simulink model "Microinverter_Paper_Model_MK_2018a"  (R2018a)
settings: Solver=FixedStepDiscrete  StartTime=0.0  StopTime=0.3  RelTol=1e-3
undefined symbols (not defined in the file): sigbuilder_block
libraries: powerlib x53, simulink x5, powerlib_meascontrol x4, re_lib x1
settings Model: Creator=jasil  LastModifiedBy=mwkane
settings SFSimCC: SimUseLocalCustomCode=on
settings RTWCC: RTWUseLocalCustomCode=on
settings CodeAppCC: StateflowObjectComments=on

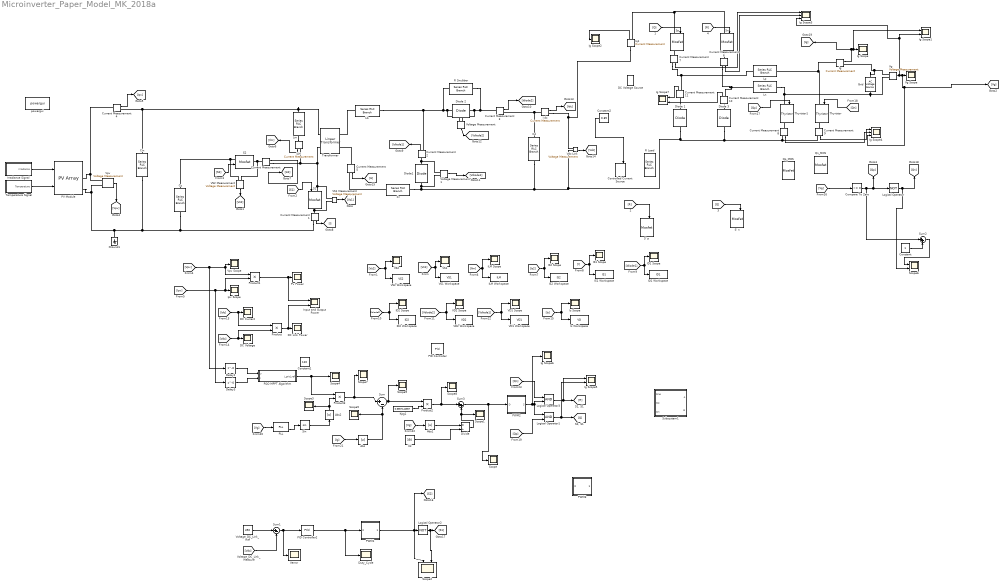
== system Microinverter_Paper_Model_MK_2018a ==
  Abs : Abs
  Abs1 : Abs
  Abs2 : Abs
  Cc : powerlib/Elements/Series RLC Branch  LConnTagsString=__new0  RConnTagsString=__new0  BranchType=RC  Resistance=0.000001  Inductance=1e-3  SetiL0=off  InitialCurrent=0  Capacitance=2.2e-6  Setx0=off  InitialVoltage=0  Measurements=None
      settings: SourceProductName=Simscape Electrical
  Cd : powerlib/Elements/Series RLC Branch  LConnTagsString=__new0  RConnTagsString=__new0  BranchType=RC  Resistance=0.000001  Inductance=1e-3  SetiL0=off  InitialCurrent=0  Capacitance=1  Setx0=off  InitialVoltage=0  Measurements=None
      settings: SourceProductName=Simscape Electrical
  Cin : powerlib/Elements/Series RLC Branch  LConnTagsString=__new0  RConnTagsString=__new0  BranchType=RC  Resistance=0.000001  Inductance=1e-3  SetiL0=off  InitialCurrent=0  Capacitance=1e-3  Setx0=off  InitialVoltage=0  Measurements=Branch voltage
      settings: SourceProductName=Simscape Electrical
  Compare To Zero : simulink/Logic and Bit Operations/Compare To Zero  relop=>=  OutDataTypeStr=boolean
  Constant : Constant
  Constant1 : Constant  Value=120
  Constant2 : Constant  Value=0.85
  Controlled Current Source : powerlib/Electrical Sources/Controlled Current Source  Initialize=on  Source_Type=AC  Amplitude=0  Phase=0  Frequency=0  Measurements=None
      settings: SourceProductName=Simscape Electrical
  Cr : powerlib/Elements/Series RLC Branch  LConnTagsString=__new0  RConnTagsString=__new0  BranchType=RC  Resistance=0.000001  Inductance=1e-3  SetiL0=off  InitialCurrent=0  Capacitance=2.4e-6  Setx0=off  InitialVoltage=0  Measurements=None
      settings: SourceProductName=Simscape Electrical
  Current Measurement{,1..11} (12 alike) : powerlib/Measurements/Current Measurement  PhasorSimulation=off  OutputType=Complex  PSBequivalent=0
      settings: SourceProductName=Simscape Electrical
  DC Current : Scope
  DC Link Power : Scope
  DC Voltage : Scope
  DC Voltage Source : powerlib/Electrical Sources/DC Voltage Source  Amplitude=350  Measurements=None
      settings: SourceProductName=Simscape Electrical
  Delay2 : Delay  DelayLength=0  SampleTime=0.0001
  Delay3 : Delay  DelayLength=0  SampleTime=0.0001
  Diode 1 : powerlib/Power Electronics/Diode  Ron=1  Lon=0  Vf=0.8  IC=0  UseSnubber=0  Rs=1e5  Cs=inf  Measurements=off
      settings: SourceProductName=Simscape Electrical
  Diode 2 : powerlib/Power Electronics/Diode  Ron=1  Lon=0  Vf=0.8  IC=0  UseSnubber=0  Rs=inf  Cs=0  Measurements=off
      settings: SourceProductName=Simscape Electrical
  Diode 3 : powerlib/Power Electronics/Diode  Ron=1  Lon=0  Vf=0.8  IC=0  UseSnubber=0  Rs=1e5  Cs=inf  Measurements=off
      settings: SourceProductName=Simscape Electrical
  Diode1 : powerlib/Power Electronics/Diode  Ron=0.01  Lon=0  Vf=0.8  IC=0  UseSnubber=0  Rs=inf  Cs=0  Measurements=off
      settings: SourceProductName=Simscape Electrical
  Divide : Product  Inputs=*/
  Duty_Cycle : Scope
  Grid : powerlib/Electrical Sources/AC Voltage Source  Amplitude=311.126  Phase=0  Frequency=60  SampleTime=0  Measurements=None  BusType=swing  Pref=0  Qref=0  Qmin=-inf  Qmax=+inf
      settings: SourceProductName=Simscape Electrical
  Ground1 : powerlib/Elements/Ground  LConnTagsString=a
      settings: SourceProductName=Simscape Electrical
  I dc : powerlib/Measurements/Current Measurement  PhasorSimulation=off  OutputType=Complex  PSBequivalent=0
      settings: SourceProductName=Simscape Electrical
  ID1 Scope : Scope
  ID1 Workspace : ToWorkspace  VariableName=ID1  SaveFormat=Timeseries  SampleTime=-1
  ID2 Scope : Scope
  ID2 Workspace : ToWorkspace  VariableName=ID2  SaveFormat=Timeseries  SampleTime=-1
  ILM Workspace : ToWorkspace  VariableName=ILM  SaveFormat=Timeseries  SampleTime=-1
  IS1 Scope : Scope
  IS1 Workspace : ToWorkspace  VariableName=IS1  SaveFormat=Timeseries  SampleTime=-1
  IS2 Scope : Scope
  IS2 Workspace : ToWorkspace  VariableName=IS2  SaveFormat=Timeseries  SampleTime=-1
  Ig : powerlib/Measurements/Current Measurement  PhasorSimulation=off  OutputType=Complex  PSBequivalent=0
      settings: SourceProductName=Simscape Electrical
  Ig Scope : Scope
  Ig Scope1 : Scope  NumInputPorts=2
  Ig Scope2 : Scope
  Ig Scope3 : Scope  NumInputPorts=3
  Ig Scope4 : Scope  NumInputPorts=3
  Ig Scope5 : Scope  NumInputPorts=2
  Ig Scope6 : Scope
  Ig Scope7 : Scope  NumInputPorts=2
  Ig1 : powerlib/Measurements/Current Measurement  PhasorSimulation=off  OutputType=Complex  PSBequivalent=0
      settings: SourceProductName=Simscape Electrical
  Input and Output Power : Scope  NumInputPorts=2
  Ipv Scope : Scope
  "Irradiance Signal " : Subsystem  Tag=STV Subsys  LoadFcn=sigbuilder_block('load');  StartFcn=sigbuilder_block('start');  StopFcn=sigbuilder_block('stop');  ClipboardFcn=sigbuilder_block('clipboard');  mask(Sigbuilder block){tuvar=[0:10]}
      mask help: Simulink:masks:SigbuilderBlock_MD
      mask init:
      | if ~strcmp(get_param(bdroot(gcbh),'SimulationStatus'),'stopped') tuvar = sigbuilder_block('maskInit'); end
      settings: CopyFcn=sigbuilder_block('copy');  DeleteFcn=sigbuilder_block('delete');  ModelCloseFcn=sigbuilder_block('modelClose');  PreSaveFcn=sigbuilder_block('preSave');  PauseFcn=sigbuilder_block('pause');  ContinueFcn=sigbuilder_block('continue');  NameChangeFcn=sigbuilder_block('namechange');  OpenFcn=sigbuilder_block('open',[6 30 1012.5 447.75 ]);  CloseFcn=sigbuilder_block('close');
      mask Display: plot(0, 0, 100, 100,[2, 2, 32, 32, 2], [68, 8, 8, 68, 68],[32, 2], [38, 38], [32, 19, 2],[53, 60, 44], [32, 17, 17, 2],[16, 16, 31, 31]);txt = getActiveGroup(gcbh);text(2, 100, txt,'verticalAlignment', 'top');
  Is Scope : Scope
  Is Workspace : ToWorkspace  VariableName=VD  SaveFormat=Timeseries  SampleTime=-1
  Kpg1 : Constant  Value=0.6857142857
  Llk : powerlib/Elements/Series RLC Branch  LConnTagsString=__new0  RConnTagsString=__new0  BranchType=RL  Resistance=0.000001  Inductance=2.6e-6  SetiL0=off  InitialCurrent=0  Capacitance=1e-6  Setx0=off  InitialVoltage=0  Measurements=None
      settings: SourceProductName=Simscape Electrical
  Lm : powerlib/Elements/Series RLC Branch  LConnTagsString=__new0  RConnTagsString=__new0  BranchType=RL  Resistance=0.000001  Inductance=20e-6  SetiL0=off  InitialCurrent=0  Capacitance=1e-6  Setx0=off  InitialVoltage=0  Measurements=None
      settings: SourceProductName=Simscape Electrical
  Ln : powerlib/Elements/Series RLC Branch  LConnTagsString=__new0  RConnTagsString=__new0  BranchType=RL  Resistance=70e-3  Inductance=15e-3  SetiL0=off  InitialCurrent=0  Capacitance=1e-6  Setx0=off  InitialVoltage=0  Measurements=None
      settings: SourceProductName=Simscape Electrical
  Logical Operator : Logic  Operator=NOT  AllPortsSameDT=off  OutDataTypeStr=boolean
  Logical Operator1 : Logic  AllPortsSameDT=off  OutDataTypeStr=boolean
  Logical Operator2 : Logic  Operator=NOT  AllPortsSameDT=off  OutDataTypeStr=boolean
  Logical Operator3 : Logic  AllPortsSameDT=off  OutDataTypeStr=boolean
  Lp : powerlib/Elements/Series RLC Branch  LConnTagsString=__new0  RConnTagsString=__new0  BranchType=RL  Resistance=70e-3  Inductance=15e-3  SetiL0=off  InitialCurrent=0  Capacitance=1e-6  Setx0=off  InitialVoltage=0  Measurements=None
      settings: SourceProductName=Simscape Electrical
  P&O MPPT Algorithm : MATLAB Function  TreatAsAtomicUnit=on
  PID Controller : simulink/Continuous/PID Controller  Controller=P  Form=Parallel  TimeDomain=Discrete-time  SampleTime=1e-6  IntegratorMethod=Forward Euler  FilterMethod=Forward Euler  ControllerParametersSource=internal  P=0.6857142857  I=1  D=0  UseFilter=on  N=100  TunerSelectOption=Transfer Function Based (PID Tuner App)  InitialConditionSource=internal  InitialConditionForIntegrator=0  InitialConditionForFilter=0  DifferentiatorICPrevScaledInput=0  ExternalReset=none  TrackingMode=off  Kt=1  LimitOutput=off  UpperSaturationLimit=1  LowerSaturationLimit=-1  LinearizeAsGain=on  AntiWindupMode=none  Kb=1  POutMin=[]  POutMax=[]  IOutMin=[]  IOutMax=[]  DOutMin=[]  DOutMax=[]  NOutMin=[]  NOutMax=[]  SumOutMin=[]  SumOutMax=[]  SaturationOutMin=[]  SaturationOutMax=[]  PParamMin=[]  PParamMax=[]  IParamMin=[]  IParamMax=[]  DParamMin=[]  DParamMax=[]  NParamMin=[]  NParamMax=[]  KbParamMin=[]  KbParamMax=[]  KtParamMin=[]  KtParamMax=[]  KbOutMin=[]  KbOutMax=[]  KtOutMin=[]  KtOutMax=[]  IntegratorOutMin=[]  IntegratorOutMax=[]  FilterOutMin=[]  FilterOutMax=[]  SumI1OutMin=[]  SumI1OutMax=[]  SumI2OutMin=[]  SumI2OutMax=[]  SumI3OutMin=[]  SumI3OutMax=[]  SumDOutMin=[]  SumDOutMax=[]  DifferentiatorOutMin=[]  DifferentiatorOutMax=[]  FilterDiffOutCoefMin=[]  FilterDiffOutCoefMax=[]  ReciprocalOutMin=[]  ReciprocalOutMax=[]  SumDenOutMin=[]  SumDenOutMax=[]  SumNumOutMin=[]  SumNumOutMax=[]  DivideOutMin=[]  DivideOutMax=[]  IntegratorContinuousStateAttributes=''  IntegratorStateMustResolveToSignalObject=off  IntegratorRTWStateStorageClass=Auto  FilterContinuousStateAttributes=''  FilterStateMustResolveToSignalObject=off  FilterRTWStateStorageClass=Auto
  PID Controller2 : simulink/Continuous/PID Controller  Controller=PI  Form=Parallel  TimeDomain=Discrete-time  SampleTime=-1  IntegratorMethod=Forward Euler  FilterMethod=Forward Euler  ControllerParametersSource=internal  P=1/3500  I=0.055  D=1  UseFilter=off  N=100  TunerSelectOption=Transfer Function Based (PID Tuner App)  InitialConditionSource=internal  InitialConditionForIntegrator=0  InitialConditionForFilter=0  DifferentiatorICPrevScaledInput=0  ExternalReset=none  TrackingMode=off  Kt=1  LimitOutput=on  UpperSaturationLimit=0.95  LowerSaturationLimit=0.05  LinearizeAsGain=on  AntiWindupMode=none  Kb=1  POutMin=[]  POutMax=[]  IOutMin=[]  IOutMax=[]  DOutMin=[]  DOutMax=[]  NOutMin=[]  NOutMax=[]  SumOutMin=[]  SumOutMax=[]  SaturationOutMin=[]  SaturationOutMax=[]  PParamMin=[]  PParamMax=[]  IParamMin=[]  IParamMax=[]  DParamMin=[]  DParamMax=[]  NParamMin=[]  NParamMax=[]  KbParamMin=[]  KbParamMax=[]  KtParamMin=[]  KtParamMax=[]  KbOutMin=[]  KbOutMax=[]  KtOutMin=[]  KtOutMax=[]  IntegratorOutMin=[]  IntegratorOutMax=[]  FilterOutMin=[]  FilterOutMax=[]  SumI1OutMin=[]  SumI1OutMax=[]  SumI2OutMin=[]  SumI2OutMax=[]  SumI3OutMin=[]  SumI3OutMax=[]  SumDOutMin=[]  SumDOutMax=[]  DifferentiatorOutMin=[]  DifferentiatorOutMax=[]  FilterDiffOutCoefMin=[]  FilterDiffOutCoefMax=[]  ReciprocalOutMin=[]  ReciprocalOutMax=[]  SumDenOutMin=[]  SumDenOutMax=[]  SumNumOutMin=[]  SumNumOutMax=[]  DivideOutMin=[]  DivideOutMax=[]  IntegratorContinuousStateAttributes=''  IntegratorStateMustResolveToSignalObject=off  IntegratorRTWStateStorageClass=Auto  FilterContinuousStateAttributes=''  FilterStateMustResolveToSignalObject=off  FilterRTWStateStorageClass=Auto
  PLL : powerlib_meascontrol/PLL/PLL  Fmin=45  Par_Init=[0, 60]  ParK=[180, 3200, 1]  TcD=1e-4  MaxRateChangeFreq=12  FilterCutOffFreq=25  Ts=1e-6  AGC=on
      settings: SourceProductName=Simscape Electrical  SourceProductBaseCode=PS
  PV Module : re_lib/Solar/PV Array  Npar=1  Nser=2  PlotType=array @ 25 deg.C & specified irradiances  S_vec="[ 1000  500  100 ]"  Temp_C_vec="[ 45 25  ]"  ModuleName=User-defined  PlotWhenSelected=off  Pm=179.9805  Ncell=36  Voc=24.06  Isc=9.77  Vm=19.67  Im=9.15  beta_Voc_pc=-0.28  alpha_Isc_pc=+0.04  beta_Voc=-0.067368  alpha_Isc=0.003908  IL=9.8911  I0=1.3829e-11  nI=0.95443  Rsh=60.4787  Rs=0.18212  BAL=off  Tc=1e-6  Tfilter=5e-5
      settings: SourceProductName=Simscape Electrical
  PWM1 : Subsystem
  PWM2 : Subsystem
  PWM3 : Subsystem
  Product{,1..3} (4 alike) : Product
  Pv Power : Scope
  Qn_MOS : powerlib/Power Electronics/Mosfet  Ron=0.1  Lon=0  Rd=0.01  Vfd=0  IC=0  Rs=1e5  Cs=inf  Measurements=on
      settings: SourceProductName=Simscape Electrical
  Qp_MOS : powerlib/Power Electronics/Mosfet  Ron=0.1  Lon=0  Rd=0.01  Vfd=0  IC=0  Rs=1e5  Cs=inf  Measurements=on
      settings: SourceProductName=Simscape Electrical
  R Load : powerlib/Elements/Series RLC Branch  LConnTagsString=__new0  RConnTagsString=__new0  BranchType=R  Resistance=695  Inductance=1e-3  SetiL0=off  InitialCurrent=0  Capacitance=1e-6  Setx0=off  InitialVoltage=0  Measurements=None
      settings: SourceProductName=Simscape Electrical
  R Snubber : powerlib/Elements/Series RLC Branch  LConnTagsString=__new0  RConnTagsString=__new0  BranchType=R  Resistance=1e6  Inductance=1e-3  SetiL0=off  InitialCurrent=0  Capacitance=1e-6  Setx0=off  InitialVoltage=0  Measurements=None
      settings: SourceProductName=Simscape Electrical
  S' n : powerlib/Power Electronics/Mosfet  Ron=0.1  Lon=0  Rd=0.01  Vfd=0  IC=0  Rs=1e5  Cs=inf  Measurements=on
      settings: SourceProductName=Simscape Electrical
  S' p : powerlib/Power Electronics/Mosfet  Ron=0.1  Lon=0  Rd=0.01  Vfd=0  IC=0  Rs=1e5  Cs=inf  Measurements=on
      settings: SourceProductName=Simscape Electrical
  S1 : powerlib/Power Electronics/Mosfet  Ron=5.6e-3  Lon=0  Rd=0.01  Vfd=1.3  IC=0  Rs=1e6  Cs=inf  Measurements=off
      settings: SourceProductName=Simscape Electrical
  S2 : powerlib/Power Electronics/Mosfet  Ron=5.6e-3  Lon=0  Rd=0.01  Vfd=1.3  IC=0  Rs=1e5  Cs=inf  Measurements=off
      settings: SourceProductName=Simscape Electrical
  Scope{,1,3..5,7..9} (8 alike) : Scope
  Scope2 : Scope  NumInputPorts=2
  Scope6 : Scope  NumInputPorts=2
  Sin : Trigonometry
  Sn : powerlib/Power Electronics/Mosfet  Ron=0.1  Lon=0  Rd=1e6  Vfd=0  IC=0  Rs=1e5  Cs=inf  Measurements=on
      settings: SourceProductName=Simscape Electrical
  Sp : powerlib/Power Electronics/Mosfet  Ron=0.1  Lon=0  Rd=1e6  Vfd=0  IC=0  Rs=1e5  Cs=inf  Measurements=on
      settings: SourceProductName=Simscape Electrical
  Subsystem1 : Subsystem
  Sum : Sum  Inputs=|+-
  Sum1 : Sum  Inputs=|+-
  Sum2 : Sum  Inputs=|++
  Sum3 : Sum  Inputs=|++
  Temperature Signal : Subsystem  Tag=STV Subsys  LoadFcn=sigbuilder_block('load');  StartFcn=sigbuilder_block('start');  StopFcn=sigbuilder_block('stop');  ClipboardFcn=sigbuilder_block('clipboard');  mask(Sigbuilder block){tuvar=[0:10]}
      mask help: Simulink:masks:SigbuilderBlock_MD
      mask init:
      | if ~strcmp(get_param(bdroot(gcbh),'SimulationStatus'),'stopped') tuvar = sigbuilder_block('maskInit'); end
      settings: CopyFcn=sigbuilder_block('copy');  DeleteFcn=sigbuilder_block('delete');  ModelCloseFcn=sigbuilder_block('modelClose');  PreSaveFcn=sigbuilder_block('preSave');  PauseFcn=sigbuilder_block('pause');  ContinueFcn=sigbuilder_block('continue');  NameChangeFcn=sigbuilder_block('namechange');  OpenFcn=sigbuilder_block('open',[6 30 1012.5 447.75 ]);  CloseFcn=sigbuilder_block('close');
      mask Display: plot(0, 0, 100, 100,[2, 2, 32, 32, 2], [68, 8, 8, 68, 68],[32, 2], [38, 38], [32, 19, 2],[53, 60, 44], [32, 17, 17, 2],[16, 16, 31, 31]);txt = getActiveGroup(gcbh);text(2, 100, txt,'verticalAlignment', 'top');
  Thyristor : powerlib/Power Electronics/Thyristor  Ron=0.1  Lon=0  Vf=0  IC=0  Rs=1e5  Cs=inf  Measurements=on
      settings: SourceProductName=Simscape Electrical
  Thyristor1 : powerlib/Power Electronics/Thyristor  Ron=0.1  Lon=0  Vf=0  IC=0  Rs=1e5  Cs=inf  Measurements=on
      settings: SourceProductName=Simscape Electrical
  Transformer : powerlib/Elements/Linear Transformer  UNITS=SI  NominalPower=[ 25 100e3 ]  winding1=[6.36 0 0]  winding2=[26.87 0 0]  ThreeWindings=off  winding3=[3.15e+05 3.969e+07 6316.9]  RmLm=[1e6 Inf]  Measurements=None  DataType=on
      settings: SourceProductName=Simscape Electrical
  VD1 Scope : Scope
  VD1 Workspace : ToWorkspace  VariableName=VD1  SaveFormat=Timeseries  SampleTime=-1
  VD2 Scope : Scope
  VD2 Workspace : ToWorkspace  VariableName=VD2  SaveFormat=Timeseries  SampleTime=-1
  VS1 : Scope
  VS1 Measurement : powerlib/Measurements/Voltage Measurement  PhasorSimulation=off  OutputType=Complex  PSBequivalent=0
      settings: SourceProductName=Simscape Electrical
  VS1 Workspace : ToWorkspace  VariableName=VS1  SaveFormat=Timeseries  SampleTime=-1
  VS2 : Scope
  VS2 Measurement : powerlib/Measurements/Voltage Measurement  PhasorSimulation=off  OutputType=Complex  PSBequivalent=0
      settings: SourceProductName=Simscape Electrical
  VS2 Workspace : ToWorkspace  VariableName=VS2  SaveFormat=Timeseries  SampleTime=-1
  Vd : Constant  Value=350
  Vdc Link : powerlib/Measurements/Voltage Measurement  PhasorSimulation=off  OutputType=Complex  PSBequivalent=0
      settings: SourceProductName=Simscape Electrical
  "Verror " : Scope
  Vg : powerlib/Measurements/Voltage Measurement  PhasorSimulation=off  OutputType=Complex  PSBequivalent=0
      settings: SourceProductName=Simscape Electrical
  Vg Scope : Scope
  Voltage Measurement : powerlib/Measurements/Voltage Measurement  PhasorSimulation=off  OutputType=Complex  PSBequivalent=0
      settings: SourceProductName=Simscape Electrical
  Voltage Measurement1 : powerlib/Measurements/Voltage Measurement  PhasorSimulation=off  OutputType=Complex  PSBequivalent=0
      settings: SourceProductName=Simscape Electrical
  Voltage_DC_Link_Ref : Constant  Value=350
  Vpv : powerlib/Measurements/Voltage Measurement  PhasorSimulation=off  OutputType=Complex  PSBequivalent=0
      settings: SourceProductName=Simscape Electrical
  Vpv Scope : Scope
  iLM : powerlib/Measurements/Current Measurement  PhasorSimulation=off  OutputType=Complex  PSBequivalent=0
      settings: SourceProductName=Simscape Electrical
  iLM Scope : Scope
  powergui : powerlib/powergui  Priority=1  SimulationMode=Discrete  SampleTime=0.9e-7  frequency=60  Iterations=50  frequencyindice=0  Pbase=100e6  ErrMax=1e-4  UnitsV=kV  UnitsW=MW  buscounter=0  FunctionMessages=off  echomessages=off  EnableUseOfTLC=off  CurrentSourceSwitches=off  DisableSnubberDevices=off  DisableRonSwitches=off  DisableVfSwitches=off  DisplayEquations=off  SolverType=Tustin/Backward Euler (TBE)  Interpol=off  ExternalGateDelay=off  methode=off  Ts=100  x0status=blocks  SPID=on  SwTol=0  HookPort=off  RestoreLinks=warning  ResistiveCurrentMeasurement=off  Frange=[0:2:500]  Ylog=off  Xlog=on  ShowGrid=off  save=off  variable=ZData  structure=0  ZoomFFT=off  StartTime=0.0  cycles=1  DisplayStyle=1  fundamental=60  FreqAxis=off  MaxFrequency=1000  frequencyindicesteady=1  RmsSteady=1  display=off
      settings: SourceProductName=Simscape Electrical
  wires:
  [Vdiode1] -> VD1 Workspace/1, VD1 Scope/1
  Vdc Link/1 -> [Vdc]
  [Vdc] -> Product/2, DC Voltage/1
  VS2 Measurement/1 -> [Vs2]
  Current Measurement1/1 -> [I]
  Vpv/1 -> [Vpv]
  Voltage Measurement/1 -> [Vdiode2]
  Voltage Measurement1/1 -> [Vdiode1]
  [S2] -> S2/1
  Current Measurement2/1 -> [Idiode1]
  [Vdiode2] -> VD2 Workspace/1, VD2 Scope/1
  [Idiode1] -> ID1 Workspace/1, ID1 Scope/1
  [Vpv] -> Delay2/1, Vpv Scope/1, Product1/1
  [Ipv] -> Delay3/1, Product1/2, Ipv Scope/1
  Current Measurement/1 -> [Is2]
  [Vs1] -> VS1 Workspace/1, VS1/1
  [S1] -> S1/1
  [I] -> IS1 Workspace/1, IS1 Scope/1
  [Vs2] -> VS2 Workspace/1, VS2/1
  iLM/1 -> [Ilm]
  Product/1 -> Input and Output Power/2, DC Link Power/1
  [Ilm] -> iLM Scope/1, ILM Workspace/1
  Delay3/1 -> P&O MPPT Algorithm/2(I)
  [Idiode2] -> ID2 Workspace/1, ID2 Scope/1
  Product1/1 -> Input and Output Power/1, Pv Power/1
  [Is2] -> IS2 Workspace/1, IS2 Scope/1
  VS1 Measurement/1 -> [Vs1]
  [Idc] -> Product/1, DC Current/1
  Delay2/1 -> P&O MPPT Algorithm/1(V)
  [Is] -> Is Workspace/1, Is Scope/1
  Current Measurement4/1 -> [Ipv]
  I dc/1 -> [Idc]
  Current Measurement3/1 -> [Idiode2]
  Current Measurement5/1 -> [Is]
  Logical Operator2/1 -> Scope2/2, [S1]
  PWM1/1(S) -> [S2], Scope2/1, Logical Operator2/1
  Voltage_DC_Link_Ref/1 -> Sum1/1
  [Vdc] -> Sum1/2
  Sum1/1 -> PID Controller2/1, "Verror "/1
  Logical Operator/1 -> Scope6/2, [Qn]
  Vg/1 -> Ig Scope3/3, Ig Scope1/2, Ig Scope4/3, [Vg], Vg Scope/1
  [R] -> Sn/1
  [Q] -> Sp/1
  [Q] -> S' n/1
  [Vg] -> Compare To Zero/1
  Ig1/1 -> Ig Scope2/1
  [R] -> S' p/1
  Constant/1 -> Sum2/2
  Compare To Zero/1 -> Sum2/1, [Qp], Logical Operator/1
  Sum2/1 -> Scope6/1
  [Vg] -> PLL/1
  PLL/2 -> Sin/1
  Product3/1 -> Scope7/1, Sum/1
  [Ig] -> Abs/1
  Vd/1 -> Divide/2
  Divide/1 -> Sum3/2, Scope1/1
  Sum3/1 -> PWM2/1(D), Scope/1
  Abs/1 -> Scope5/1, Sum/2
  [Vg] -> Abs1/1
  Abs1/1 -> Divide/1
  Current Measurement7/1 -> Ig Scope3/1
  Current Measurement6/1 -> Ig Scope3/2
  Sin/1 -> Abs2/1
  Abs2/1 -> Product3/2, Scope3/1
  PWM2/1(S) -> Ig Scope6/1, Logical Operator3/2, Logical Operator1/1
  Logical Operator1/1 -> Ig Scope5/2, [Q]
  Logical Operator3/1 -> Ig Scope5/1, [R]
  [Qp] -> Logical Operator1/2
  [Qn] -> Logical Operator3/1
  Current Measurement9/1 -> Ig Scope4/1
  Current Measurement8/1 -> Ig Scope4/2
  Sum/1 -> Product2/1, Scope9/1
  PID Controller2/1 -> PWM1/1(D), Duty_Cycle/1
  Constant2/1 -> Controlled Current Source/1
  [Qn] -> Thyristor/1
  [Qp] -> Thyristor1/1
  Current Measurement11/1 -> Ig Scope7/1
  Current Measurement10/1 -> Ig Scope7/2
  Ig/1 -> [Ig], Ig Scope1/1, Ig Scope/1
  Product2/1 -> Scope8/1, Sum3/1
  Kpg1/1 -> Product2/2
  P&O MPPT Algorithm/1(I_grid_ref) -> Product3/1, Scope4/1
  "Irradiance Signal "/1(Irradiance) -> PV Module/1
  Temperature Signal/1(Temperature) -> PV Module/2
  connections:
  Current Measurement1/RConn1 -- PV Module/RConn2 -- Vpv/LConn2 -- Ground1/LConn1 -- Cin/RConn1 -- Cc/RConn1
  Llk/RConn1 -- R Snubber/LConn1 -- Voltage Measurement/LConn2 -- Diode 2/LConn1 -- Current Measurement2/RConn1
  VS1 Measurement/LConn2 -- Current Measurement1/LConn1 -- S1/RConn1
  S2/LConn1 -- VS2 Measurement/LConn1 -- Cc/LConn1
  iLM/RConn1 -- S1/LConn1 -- VS1 Measurement/LConn1 -- Transformer/LConn2 -- Current Measurement/RConn1
  Cd/LConn1 -- I dc/LConn1 -- Current Measurement3/RConn1
  S2/RConn1 -- VS2 Measurement/LConn2 -- Current Measurement/LConn1
  Lm/RConn1 -- iLM/LConn1
  Cr/LConn1 -- Current Measurement5/RConn1
  I dc/RConn1 -- Ig1/LConn1 -- Vdc Link/LConn1
  Lm/LConn1 -- Cin/LConn1 -- Current Measurement4/RConn1 -- Transformer/LConn1
  Vpv/LConn1 -- PV Module/RConn1 -- Current Measurement4/LConn1
  Diode 2/RConn1 -- Voltage Measurement/LConn1 -- R Snubber/RConn1 -- Current Measurement3/LConn1
  Diode1/RConn1 -- Voltage Measurement1/LConn1 -- Current Measurement2/LConn1
  Vg/LConn1 -- Grid/RConn1 -- Ig/RConn1
  Current Measurement7/RConn1 -- Current Measurement11/RConn1 -- Lp/LConn1
  Ln/RConn1 -- Thyristor1/LConn1 -- Grid/LConn1 -- Vg/LConn2
  Current Measurement6/RConn1 -- Current Measurement10/RConn1 -- Ln/LConn1
  Thyristor/LConn1 -- Ig/LConn1 -- Lp/RConn1
  Sn/LConn1 -- Ig1/RConn1 -- Sp/LConn1
  Current Measurement6/LConn1 -- Sn/RConn1
  Current Measurement7/LConn1 -- Sp/RConn1
  Current Measurement8/LConn1 -- Thyristor1/RConn1
  Current Measurement9/LConn1 -- Thyristor/RConn1
  Diode 3/LConn1 -- Vdc Link/LConn2 -- Cr/RConn1 -- Voltage Measurement1/LConn2 -- Diode1/LConn1 -- Cd/RConn1 -- Diode 1/LConn1 -- Current Measurement9/RConn1 -- Current Measurement8/RConn1
  Llk/LConn1 -- Transformer/RConn1
  Current Measurement5/LConn1 -- Transformer/RConn2
  Diode 3/RConn1 -- Current Measurement10/LConn1
  Diode 1/RConn1 -- Current Measurement11/LConn1

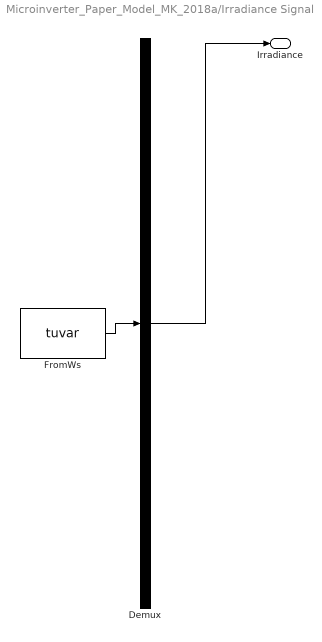
== system Microinverter_Paper_Model_MK_2018a/Irradiance Signal  ==
  Demux : Demux  Tag=STV Demux  Outputs=1
  FromWs : FromWorkspace  Tag=STV FromWs  VariableName=tuvar  SampleTime=0
      SigBuilderData=|
      | common.afterFinalStr = 'Extrapolate'
      | common.sampleTime = 0
      | dataSet.timeRange = [0 0.3]
      | dataSet.name = 'Group 1'
      | sbobj.Groups.Name = 'Group 1'
      | sbobj.Groups.Signals.Name = 'Irradiance'
      | sbobj.Groups.Signals.XData = [0 0.1 0.2 0.3]
      | sbobj.Groups.Signals.YData = [1000 1000 1000 1000]
      | sbobj.Groups.TimeRange = [0 0.3]
  Irradiance : Outport  Tag=STV Outport
  wires:
  Demux/1 -> Irradiance/1
  FromWs/1 -> Demux/1

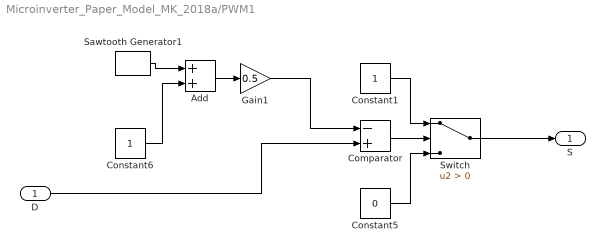
== system Microinverter_Paper_Model_MK_2018a/PWM1 ==
  D : Inport
  Add : Sum
  Comparator : Sum  Inputs=-+
  Constant1 : Constant
  Constant5 : Constant  Value=0
  Constant6 : Constant
  Gain1 : Gain  Gain=0.5
  Sawtooth Generator1 : powerlib_meascontrol/Pulse & Signal Generators/Sawtooth Generator  Freq=50000  Phase=180  Ts=0
      settings: SourceProductName=Simscape Electrical
  Switch : Switch  Criteria=u2 > Threshold
  S : Outport
  wires:
  Switch/1 -> S/1
  Constant1/1 -> Switch/1
  Comparator/1 -> Switch/2
  Constant6/1 -> Add/2
  Gain1/1 -> Comparator/1
  Constant5/1 -> Switch/3
  Sawtooth Generator1/1 -> Add/1
  Add/1 -> Gain1/1
  D/1 -> Comparator/2

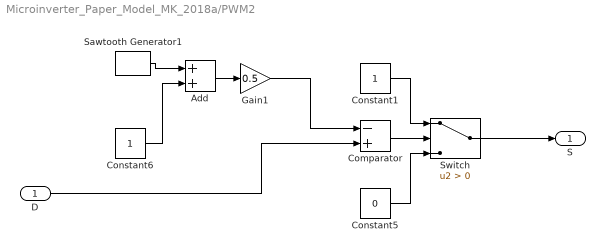
== system Microinverter_Paper_Model_MK_2018a/PWM2 ==
  D : Inport
  Add : Sum
  Comparator : Sum  Inputs=-+
  Constant1 : Constant
  Constant5 : Constant  Value=0
  Constant6 : Constant
  Gain1 : Gain  Gain=0.5
  Sawtooth Generator1 : powerlib_meascontrol/Pulse & Signal Generators/Sawtooth Generator  Freq=16000  Phase=180  Ts=0
      settings: SourceProductName=Simscape Electrical
  Switch : Switch  Criteria=u2 > Threshold
  S : Outport
  wires:
  Switch/1 -> S/1
  Constant1/1 -> Switch/1
  Comparator/1 -> Switch/2
  Constant6/1 -> Add/2
  Gain1/1 -> Comparator/1
  Constant5/1 -> Switch/3
  Sawtooth Generator1/1 -> Add/1
  Add/1 -> Gain1/1
  D/1 -> Comparator/2

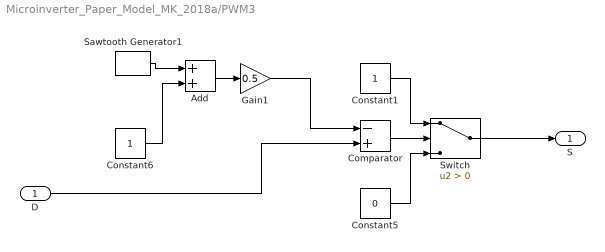
== system Microinverter_Paper_Model_MK_2018a/PWM3 ==
  D : Inport
  Add : Sum
  Comparator : Sum  Inputs=-+
  Constant1 : Constant
  Constant5 : Constant  Value=0
  Constant6 : Constant
  Gain1 : Gain  Gain=0.5
  Sawtooth Generator1 : powerlib_meascontrol/Pulse & Signal Generators/Sawtooth Generator  Freq=16000  Phase=180  Ts=0
      settings: SourceProductName=Simscape Electrical
  Switch : Switch  Criteria=u2 > Threshold
  S : Outport
  wires:
  Switch/1 -> S/1
  Constant1/1 -> Switch/1
  Comparator/1 -> Switch/2
  Constant6/1 -> Add/2
  Gain1/1 -> Comparator/1
  Constant5/1 -> Switch/3
  Sawtooth Generator1/1 -> Add/1
  Add/1 -> Gain1/1
  D/1 -> Comparator/2

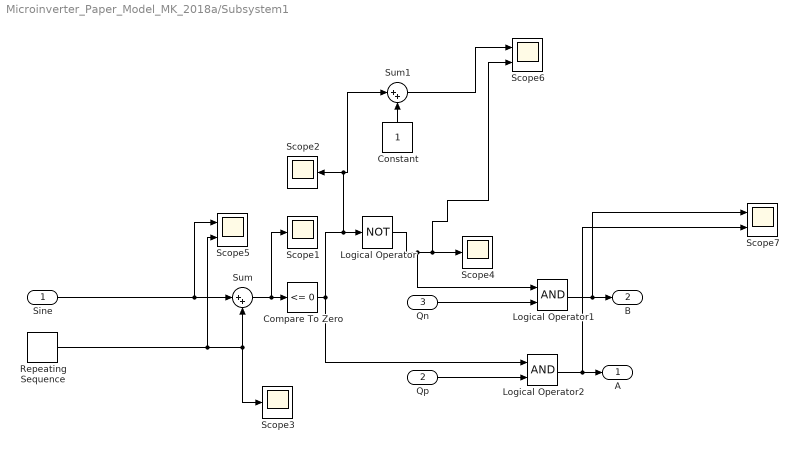
== system Microinverter_Paper_Model_MK_2018a/Subsystem1 ==
  Sine : Inport
  Qp : Inport  Port=2
  Qn : Inport  Port=3
  Compare To Zero : simulink/Logic and Bit Operations/Compare To Zero  relop=<=  OutDataTypeStr=boolean
  Constant : Constant
  Logical Operator : Logic  Operator=NOT  AllPortsSameDT=off  OutDataTypeStr=boolean
  Logical Operator1 : Logic  AllPortsSameDT=off  OutDataTypeStr=boolean
  Logical Operator2 : Logic  AllPortsSameDT=off  OutDataTypeStr=boolean
  Repeating Sequence : simulink/Sources/Repeating Sequence  rep_seq_t=[0 1/(4*16000) 3/(4*16000) 1/16000]  rep_seq_y=[0 1 -1 0]
  Scope{1..4} (4 alike) : Scope
  Scope5 : Scope  NumInputPorts=2
  Scope6 : Scope  NumInputPorts=2
  Scope7 : Scope  NumInputPorts=2
  Sum : Sum  Inputs=|++
  Sum1 : Sum  Inputs=|++
  A : Outport
  B : Outport  Port=2
  wires:
  Logical Operator/1 -> Logical Operator1/1, Scope6/2, Scope4/1
  Sum/1 -> Scope1/1, Compare To Zero/1
  Repeating Sequence/1 -> Scope5/2, Scope3/1, Sum/2
  Sine/1 -> Scope5/1, Sum/1
  Compare To Zero/1 -> Logical Operator2/1, Sum1/1, Scope2/1, Logical Operator/1
  Constant/1 -> Sum1/2
  Sum1/1 -> Scope6/1
  Logical Operator1/1 -> Scope7/1, B/1
  Logical Operator2/1 -> Scope7/2, A/1
  Qp/1 -> Logical Operator2/2
  Qn/1 -> Logical Operator1/2

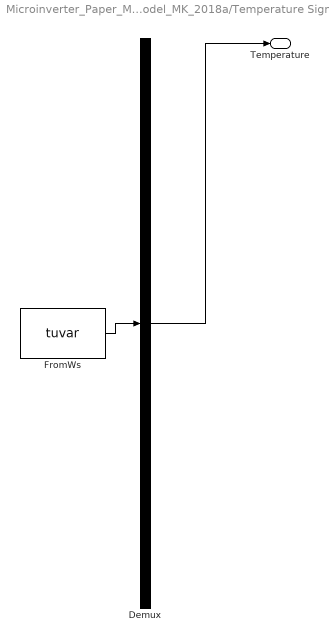
== system Microinverter_Paper_Model_MK_2018a/Temperature Signal ==
  Demux : Demux  Tag=STV Demux  Outputs=1
  FromWs : FromWorkspace  Tag=STV FromWs  VariableName=tuvar  SampleTime=0
      SigBuilderData=|
      | common.afterFinalStr = 'Extrapolate'
      | common.sampleTime = 0
      | dataSet.timeRange = [0 0.3]
      | dataSet.name = 'Group 1'
      | sbobj.Groups.Name = 'Group 1'
      | sbobj.Groups.Signals.Name = 'Temperature'
      | sbobj.Groups.Signals.XData = [0 0.1 0.2 0.3]
      | sbobj.Groups.Signals.YData = [25 25 25 25]
      | sbobj.Groups.TimeRange = [0 0.3]
  Temperature : Outport  Tag=STV Outport
  wires:
  Demux/1 -> Temperature/1
  FromWs/1 -> Demux/1

== matlab function Microinverter_Paper_Model_MK_2018a/P&O MPPT Algorithm ==
  data: V input; I_grid_ref output; I input
% function D = PandO(V, I)
% persistent p_prev;
% persistent v_prev;
% persistent d_prev; 
% 
% 
% if isempty(d_prev)
%     d_prev = 0.69;
%     v_prev = 24.06;
%     p_prev = 0;
% end
% 
% % Select the change in duty cycle
% delta_D = 0.001;
% 
% % Set local variables and calculate pv module power 
% Vn = V;
% In = I;
% Pn = Vn*In;
% 
% % Increase or decrease duty cycle based on conditions
% if ((Pn - p_prev) ~= 0)
%     if ((Pn - p_prev) > 0)
%         if ((Vn - v_prev) > 0)
%             D = d_prev - delta_D;
%         else
%             D = d_prev + delta_D;
%         end
%     else
%         if ((Vn - v_prev) > 0)
%             D = d_prev + delta_D;
%         else
%             D = d_prev - delta_D;
%         end        
%     end
% else
%     D = d_prev;
% end
% 
% % Update internal values
% d_prev = D;
% v_prev = Vn;
% p_prev = Pn;

function I_grid_ref = fcn(V,I)

persistent Vprev Pprev Iprev;

if isempty(Vprev)
    Vprev=30;
    Pprev=0;
    Iprev=0;
end

deltaI=1;

P = V * I;
    if (P>Pprev)
        if V > Vprev
            I_grid_ref = Iprev + deltaI;
        else
            I_grid_ref = Iprev - deltaI;
        end
    else
        if V > Vprev
            I_grid_ref = Iprev - deltaI;
        else
            I_grid_ref = Iprev + deltaI;
        end
    end
Vprev = V;
Pprev = P;
Iprev = I_grid_ref;

end
